simulink model "armMajorUse"  (R2023b)
settings: Solver=VariableStepAuto  StartTime=0.0  StopTime=inf  RelTol=1e-3
undefined symbols (not defined in the file): Ts
libraries: dxlSimLibrary x7
settings Model: Creator=tyler  LastModifiedBy=Tyler J

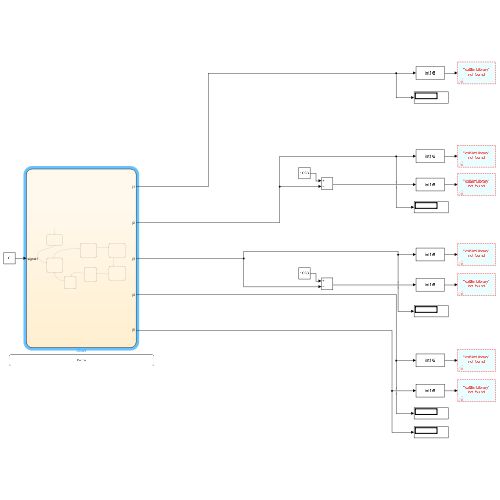
[thumbnail: Simulink's stored preview of the top-level diagram]
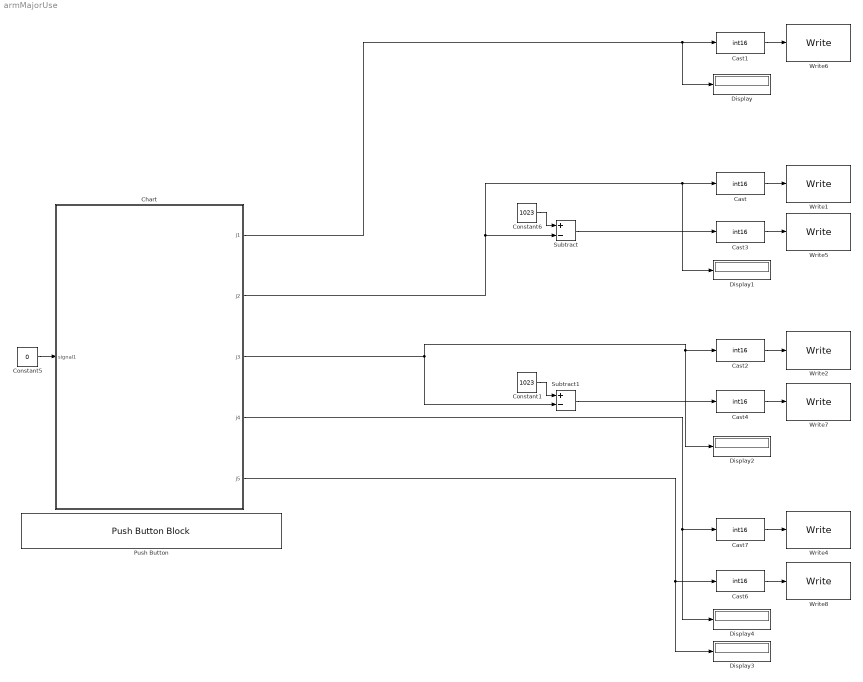
== system armMajorUse ==
  Cast{,1..4,6..7} (7 alike) : DataTypeConversion  OutDataTypeStr=int16  SaturateOnIntegerOverflow=off  RndMeth=Floor
  Chart : Stateflow chart  TreatAsAtomicUnit=on
  Constant1 : Constant  Value=1023
  Constant5 : Constant  Value=0
  Constant6 : Constant  Value=1023
  Display{,1..4} (5 alike) : Display
  Push Button : PushButtonBlock  OffValue=0.000000
  Subtract : Sum  Inputs=+-
  Subtract1 : Sum  Inputs=+-
  Write1 : dxlSimLibrary/Write  Description=|  lib_name=lib_name  port_num=port_num  protocol_version=protocol_version  ids=2  models=motor_models  select=Goal Position  Ts=Ts
      | Dynamixel library for Matlab and Simulink
      | Write function
      | Author: Georgios Andrikopoulos (geoand@kth.se), 2022 
      | Mechatronics & Embedded Control Systems Unit, KTH, Stockholm
  Write2 : dxlSimLibrary/Write  Description=|  lib_name=lib_name  port_num=port_num  protocol_version=protocol_version  ids=4  models=motor_models  select=Goal Position  Ts=Ts
      | Dynamixel library for Matlab and Simulink
      | Write function
      | Author: Georgios Andrikopoulos (geoand@kth.se), 2022 
      | Mechatronics & Embedded Control Systems Unit, KTH, Stockholm
  Write4 : dxlSimLibrary/Write  Description=|  lib_name=lib_name  port_num=port_num  protocol_version=protocol_version  ids=6  models=motor_models  select=Goal Position  Ts=Ts
      | Dynamixel library for Matlab and Simulink
      | Write function
      | Author: Georgios Andrikopoulos (geoand@kth.se), 2022 
      | Mechatronics & Embedded Control Systems Unit, KTH, Stockholm
  Write5 : dxlSimLibrary/Write  Description=|  lib_name=lib_name  port_num=port_num  protocol_version=protocol_version  ids=3  models=motor_models  select=Goal Position  Ts=Ts
      | Dynamixel library for Matlab and Simulink
      | Write function
      | Author: Georgios Andrikopoulos (geoand@kth.se), 2022 
      | Mechatronics & Embedded Control Systems Unit, KTH, Stockholm
  Write6 : dxlSimLibrary/Write  Description=|  lib_name=lib_name  port_num=port_num  protocol_version=protocol_version  ids=1  models=motor_models  select=Goal Position  Ts=Ts
      | Dynamixel library for Matlab and Simulink
      | Write function
      | Author: Georgios Andrikopoulos (geoand@kth.se), 2022 
      | Mechatronics & Embedded Control Systems Unit, KTH, Stockholm
  Write7 : dxlSimLibrary/Write  Description=|  lib_name=lib_name  port_num=port_num  protocol_version=protocol_version  ids=5  models=motor_models  select=Goal Position  Ts=Ts
      | Dynamixel library for Matlab and Simulink
      | Write function
      | Author: Georgios Andrikopoulos (geoand@kth.se), 2022 
      | Mechatronics & Embedded Control Systems Unit, KTH, Stockholm
  Write8 : dxlSimLibrary/Write  Description=|  lib_name=lib_name  port_num=port_num  protocol_version=protocol_version  ids=7  models=motor_models  select=Goal Position  Ts=Ts
      | Dynamixel library for Matlab and Simulink
      | Write function
      | Author: Georgios Andrikopoulos (geoand@kth.se), 2022 
      | Mechatronics & Embedded Control Systems Unit, KTH, Stockholm
  wires:
  Constant5/1 -> Chart/1(signal1)
  Cast/1 -> Write1/1
  Cast1/1 -> Write6/1
  Cast3/1 -> Write5/1
  Cast7/1 -> Write4/1
  Cast2/1 -> Write2/1
  Cast4/1 -> Write7/1
  Constant6/1 -> Subtract/1
  Cast6/1 -> Write8/1
  Chart/1(j1) -> Cast1/1, Display/1
  Chart/2(j2) -> Display1/1, Cast/1, Subtract/2
  Subtract/1 -> Cast3/1
  Chart/3(j3) -> Display2/1, Cast2/1, Subtract1/2
  Chart/4(j4) -> Display4/1, Cast7/1
  Chart/5(j5) -> Display3/1, Cast6/1
  Constant1/1 -> Subtract1/1
  Subtract1/1 -> Cast4/1

== stateflow chart armMajorUse/Chart ==
  state Initialize
    j1 = 512;
    j2 = 512;
    j3 = 512;
    j4 = 512;
    j5 = 800;
  state MovingToPositionCar
    j1 = 512;
    j2 = 512-80;
    j3 = 512-400;
    j4 = 512;
    j5 = 800;
  state CloseEE
    j1 = 512;
    j2 = 512-80;
    j3 = 512-400;
    j4 = 512;
    j5 = 1000;
  state RaiseArm
    j1 = 512;
    j2 = 512-150;
    j3 = 512;
    j4 = 512;
    j5 = 800;
  state RaiseArm2
    j1 = 512;
    j2 = 512-150;
    j3 = 512;
    j4 = 512;
    j5 = 1000;
  state StateDownBelt
    j1 = 512+(300);
    j2 = 512-110;
    j3 = 512-400;
    j4 = 512;
    j5 = 1000;
  state OpenEE
    j1 = 512+(300);
    j2 = 512-110;
    j3 = 512-400;
    j4 = 512;
    j5 = 800;
  (default) -> Initialize
  Initialize -> RaiseArm : [signal1>0]
  MovingToPositionCar -> CloseEE : after(0.25, sec)
  RaiseArm -> MovingToPositionCar : [signal1>0]
  CloseEE -> RaiseArm2 : [after(0.25,sec)]
  OpenEE -> RaiseArm : [after(0.25,sec)]
  StateDownBelt -> OpenEE : [after(0.25,sec)]
  RaiseArm2 -> StateDownBelt : [signal1>0]
  data: j1 output; j2 output; j3 output; j4 output; j5 output; signal1 input
